simulink model "Testing_Image_Acquire"  (R2019a)
settings: Solver=FixedStepAuto  StartTime=0.1  StopTime=0.4  FixedStep=0.001  RelTol=1e-3
values from neighbouring files (symbols this model uses):
  Epiphan_speed = round(1/Epiphan_speed,3)    [Simulink_Image_Acq_V2.m]    (also in Testing_Script.m)
undefined symbols (not defined in the file or in its folder): none, videoinput
libraries: imaqlib x1
settings Model: EnablePacing=on  Creator=asgar  LastModifiedBy=David
settings DataIOCC: ReturnWorkspaceOutputs=off
settings DebuggingCC: ArithmeticOperatorsInVariantConditions=warning

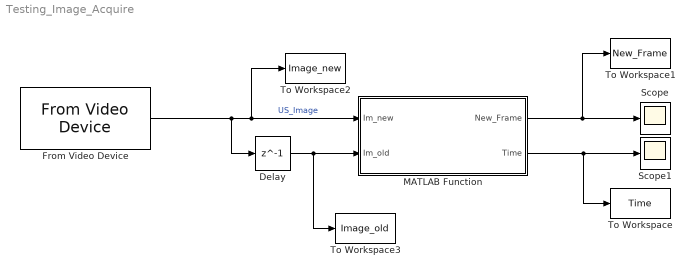
== system Testing_Image_Acquire ==
  Delay : Delay  DelayLength=1  InputProcessing=Columns as channels (frame based)  SampleTime=Epiphan_speed
  From Video Device : imaqlib/From Video Device  DeviceMenu=winvideo 1 (DVI2USB 3.0 D2S300156)  Device=winvideo 1 (DVI2USB 3.0 D2S300156)  ObjConstructor=videoinput('winvideo', 1)  VideoFormatMenu=RGB565_1280x1024  VideoFormat=RGB565_1280x1024  VideoSource=input1  ROIPosition=[107 366 783 395]  EnableHWTrigger=off  TriggerConfiguration=none/none  SampleTime=0.017  OutputPortsMode=One multidimensional signal  DataType=single  CanDoHWTrigger=no  ReturnedColorSpace=grayscale  BlockHandle=4090.0001  ROIWidth=395  ROIHeight=783  ROIColumn=366  ROIRow=107  EngXMLPath=C:\Program Files\MATLAB\R2019a\toolbox\imaq\imaq\private  DevXMLPath=C:\ProgramData\MATLAB\SupportPackages\R2019a\toolbox\imaq\supportpackages\genericvideo\adaptor\win64  EngLibPath=C:\Program Files\MATLAB\R2019a\toolbox\imaq\imaqblks\imaqmex\win64  ColorSpace=grayscale  BayerSensorAlignment=grbg  ImaqMode=off
      settings: SourceProductName=Image Acquisition Toolbox
  MATLAB Function : MATLAB Function  TreatAsAtomicUnit=on
  Scope : Scope
  Scope1 : Scope
  To Workspace : ToWorkspace  VariableName=Time  SampleTime=-1
      settings: Save2DSignal=2-D array (concatenate along first dimension)
  To Workspace1 : ToWorkspace  VariableName=New_Frame  SampleTime=-1
      settings: Save2DSignal=2-D array (concatenate along first dimension)
  To Workspace2 : ToWorkspace  VariableName=Image_new  SaveFormat=Structure  SampleTime=-1
  To Workspace3 : ToWorkspace  VariableName=Image_old  SaveFormat=Structure  SampleTime=-1
  wires:
  From Video Device/1 -> To Workspace2/1, MATLAB Function/1(Im_new), Delay/1  "US_Image"
  Delay/1 -> To Workspace3/1, MATLAB Function/2(Im_old)
  MATLAB Function/1(New_Frame) -> To Workspace1/1, Scope/1
  MATLAB Function/2(Time) -> To Workspace/1, Scope1/1

== matlab function Testing_Image_Acquire/MATLAB Function ==
  data: Im_new input; New_Frame output; Im_old input; Time output
function [New_Frame,Time] = New_Frame(Im_new,Im_old)
tic; % Starting timer

% square_dim = [1 1 783-1 395-1];
% 
% Im_new = Im_new(square_dim(1):square_dim(1)+square_dim(3),...
%     square_dim(2):square_dim(1)+square_dim(4));
% Im_old = Im_old(square_dim(1):square_dim(1)+square_dim(3),...
%     square_dim(2):square_dim(1)+square_dim(4));

if any(sum(sum(Im_old))) && any(sum(sum(Im_new)))
    same = sum(sum(Im_new - Im_old));
    New_Frame = any(same);
else
    New_Frame = false;
end

Image = cell(1,2);
Image{1} = Im_old;
Image{2} = Im_new;

Time = toc;

% function [New_Frame,Time] = New_Frame(Im_new,Im_old)
% tic; % Starting timer
%
% square_dim = [1 1 783-1 395-1];
%
% crop_Im_new = Im_new(square_dim(1):square_dim(1)+square_dim(3),...
%     square_dim(2):square_dim(1)+square_dim(4));
% crop_Im_old = Im_old(square_dim(1):square_dim(1)+square_dim(3),...
%     square_dim(2):square_dim(1)+square_dim(4));
%
% if any(sum(sum(crop_Im_old))) && any(sum(sum(crop_Im_new)))
%     same = sum(sum(crop_Im_new - crop_Im_old));
%     New_Frame = any(same);
% else
%     New_Frame = false;
% end
%
% Time = toc;
